simulink model "chap7_03_FLC_Simulink"  (R2017a)
settings: Solver=FixedStepDiscrete  StartTime=0.0  StopTime=1500  RelTol=1e-3
libraries: fuzblock x1
settings Model: Creator=Administrator  LastModifiedBy=Administrator

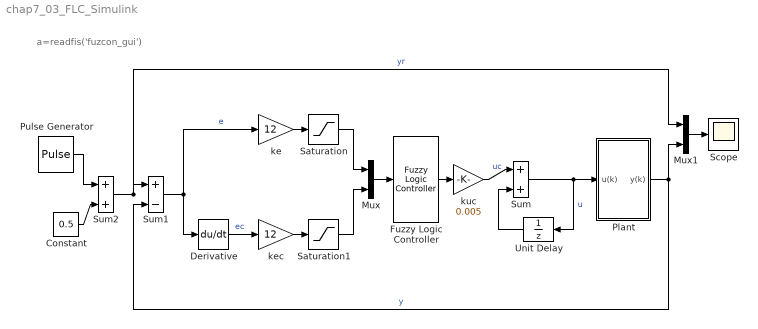
== system chap7_03_FLC_Simulink ==
  note: a=readfis('fuzcon_gui')
  Constant : Constant  Value=0.5
  Derivative : Derivative
  Fuzzy Logic Controller : fuzblock/Fuzzy Logic  Controller  fis=a
  Mux : Mux  Inputs=2
  Mux1 : Mux  Inputs=2
  Plant : Subsystem
  Pulse Generator : DiscretePulseGenerator  Amplitude=0.5  Period=1000  PulseWidth=500
  Saturation : Saturate  UpperLimit=6  LowerLimit=-6
  Saturation1 : Saturate  UpperLimit=6  LowerLimit=-6
  Scope : Scope
  Sum : Sum  Inputs=|++
  Sum1 : Sum  Inputs=|+-
  Sum2 : Sum  Inputs=|++
  Unit Delay : UnitDelay
  ke : Gain  Gain=12
  kec : Gain  Gain=12
  kuc : Gain  Gain=0.005
  wires:
  Saturation/1 -> Mux/1
  Constant/1 -> Sum2/2
  Sum2/1 -> Sum1/1, Mux1/1  "yr"
  Pulse Generator/1 -> Sum2/1
  Unit Delay/1 -> Sum/2
  Sum1/1 -> Derivative/1, ke/1  "e"
  kuc/1 -> Sum/1  "uc"
  Derivative/1 -> kec/1  "ec"
  Mux/1 -> Fuzzy Logic Controller/1
  Plant/1(y(k)) -> Mux1/2, Sum1/2  "y"
  kec/1 -> Saturation1/1
  Fuzzy Logic Controller/1 -> kuc/1
  ke/1 -> Saturation/1
  Sum/1 -> Plant/1(u(k)), Unit Delay/1  "u"
  Saturation1/1 -> Mux/2
  Mux1/1 -> Scope/1

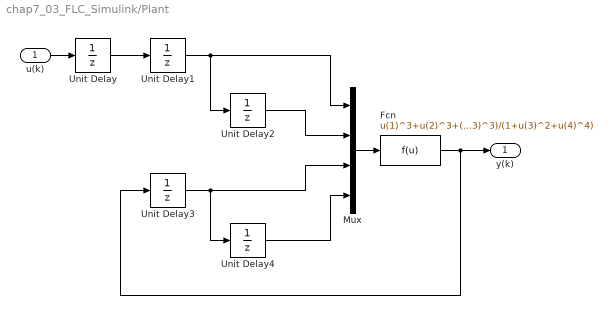
== system chap7_03_FLC_Simulink/Plant ==
  u(k) : Inport
  Fcn : Fcn  Expr=u(1)^3+u(2)^3+(0.8+u(3)^3)/(1+u(3)^2+u(4)^4)
  Mux : Mux
  Unit Delay{,1..4} (5 alike) : UnitDelay
  y(k) : Outport
  wires:
  Unit Delay/1 -> Unit Delay1/1
  Unit Delay1/1 -> Mux/1, Unit Delay2/1
  Unit Delay2/1 -> Mux/2
  Unit Delay3/1 -> Mux/3, Unit Delay4/1
  Unit Delay4/1 -> Mux/4
  Mux/1 -> Fcn/1
  u(k)/1 -> Unit Delay/1
  Fcn/1 -> y(k)/1, Unit Delay3/1
